simulink subsystem "frontierdemo_subsystem"  (R2025b)
settings: Solver=VariableStepAuto  StartTime=0.0  StopTime=10.0  RelTol=1e-3
settings Model: Creator=sanborkl  LastModifiedBy=sanborkl

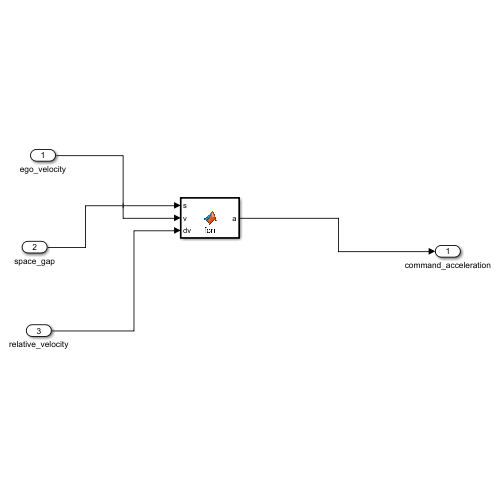
[thumbnail: Simulink's stored preview of the top-level diagram]
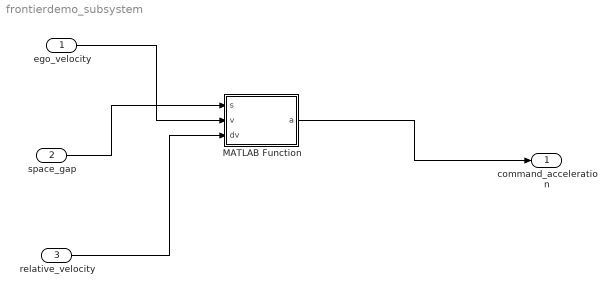
== system frontierdemo_subsystem ==
  ego_velocity : Inport
  space_gap : Inport  Port=2
  relative_velocity : Inport  Port=3
  MATLAB Function : MATLAB Function  TreatAsAtomicUnit=on
  command_acceleration : Outport
  wires:
  ego_velocity/1 -> MATLAB Function/2(v)
  space_gap/1 -> MATLAB Function/1(s)
  relative_velocity/1 -> MATLAB Function/3(dv)
  MATLAB Function/1(a) -> command_acceleration/1

== matlab function frontierdemo_subsystem/MATLAB Function ==
  data: s input; a output; v input; dv input
function a = fcn(s, v, dv)

tau = 3.0;

dmin = 10.0;

k1 = (1 / tau);

k2 = 0.25;

a = k1(k2(s - (tau * v + dmin)) + dv);
